simulink model "echo_effet"  (R2019a)
settings: Solver=VariableStepAuto  StartTime=0.0  StopTime=120  RelTol=1e-3
libraries: Librairie x2, dspobslib x1
settings Model: Creator=Ahmed  LastModifiedBy=Ahmed

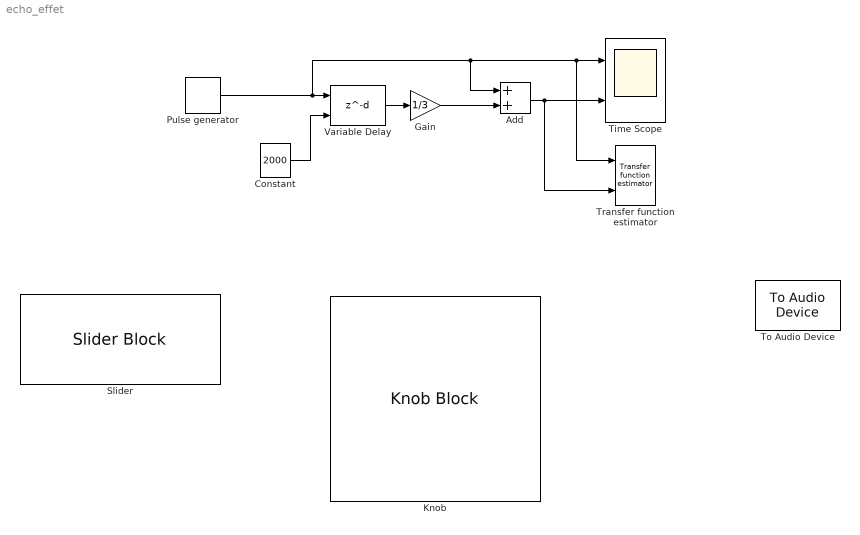
== system echo_effet ==
  Add : Sum
  Constant : Constant  Value=2000  VectorParams1D=off
  Gain : Gain  Gain=1/3
  Knob : KnobBlock  ScaleMax=96000
  Pulse generator : Librairie/Pulse generator  fee=11025  NN=1024
  Slider : SliderBlock  ScaleMax=1
  Time Scope : Scope  NumInputPorts=2
  To Audio Device : dspobslib/To Audio Device  deviceName=Default  inheritSampleRate=on  sampleRate=44100  deviceDatatype=Determine from input data type  autoBufferSize=on  bufferSize=4096  queueDuration=1.0  defaultOutputChannelMapping=on  outputChannelMapping=1:2  outputNumUnderrunSamples=off
      settings: SourceProductName=DSP System Toolbox  SourceProductBaseCode=DS
  Transfer function estimator : Librairie/Transfer function estimator  fee=11025  NN=1024
  Variable Delay : Delay  DelayLengthSource=Input port  DelayLength=1  DelayLengthUpperLimit=5000  PreventDirectFeedthrough=on  RemoveDelayLengthCheckInGeneratedCode=on  InputProcessing=Columns as channels (frame based)
      settings: InputPortMap=u0,p1
  wires:
  Add/1 -> Transfer function estimator/2, Time Scope/2
  Pulse generator/1 -> Transfer function estimator/1, Time Scope/1, Add/1, Variable Delay/1
  Gain/1 -> Add/2
  Variable Delay/1 -> Gain/1
  Constant/1 -> Variable Delay/2
